simulink model "bldc_2016_mamf"  (R2016b)
settings: Solver=FixedStepAuto  StartTime=0.0  StopTime=t_max  FixedStep=timestep  RelTol=1e-3
values from neighbouring files (symbols this model uses):
  den = [(L*J) (L*D+R*J) Kt*Kb]    [script.m]
  num = Kt*Kb    (= 0.02053489)    [script.m]
  step_v = 1000    [script.m]
settings Model: Creator=ricar  LastModifiedBy=Gabriel

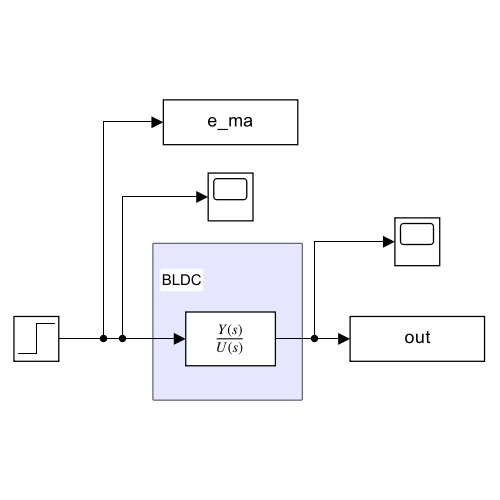
[thumbnail: Simulink's stored preview of the top-level diagram]
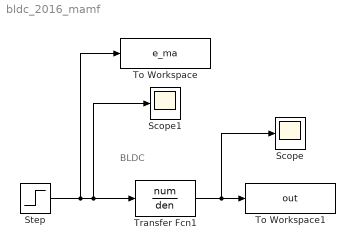
== system bldc_2016_mamf ==
  note: BLDC
  Scope : Scope
  Scope1 : Scope
  Step : Step  Time=0  After=step_v  SampleTime=0
  To Workspace : ToWorkspace  VariableName=e_ma  SampleTime=-1
  To Workspace1 : ToWorkspace  VariableName=out  SampleTime=-1
  Transfer Fcn1 : TransferFcn  Numerator=num  Denominator=den
  wires:
  Step/1 -> Transfer Fcn1/1, Scope1/1, To Workspace/1
  Transfer Fcn1/1 -> To Workspace1/1, Scope/1
